simulink model "two_cell_balancing"  (R2024b)
settings: Solver=VariableStepAuto  StartTime=0.0  StopTime=3600  RelTol=1e-3
libraries: simulink x7
settings Model: Creator=nirmithpuneet  LastModifiedBy=nirmithpuneet
settings DebuggingCC: AlgebraicLoopMsg=none

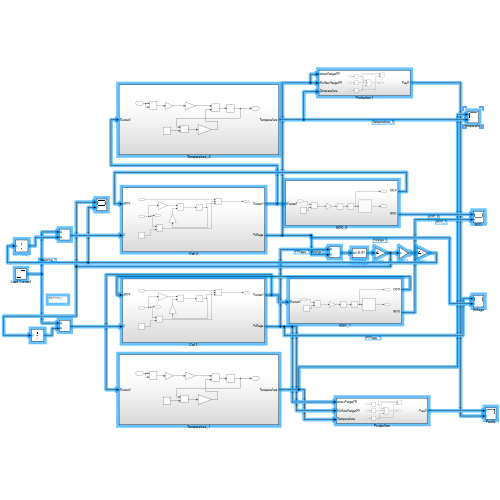
[thumbnail: Simulink's stored preview of the top-level diagram]
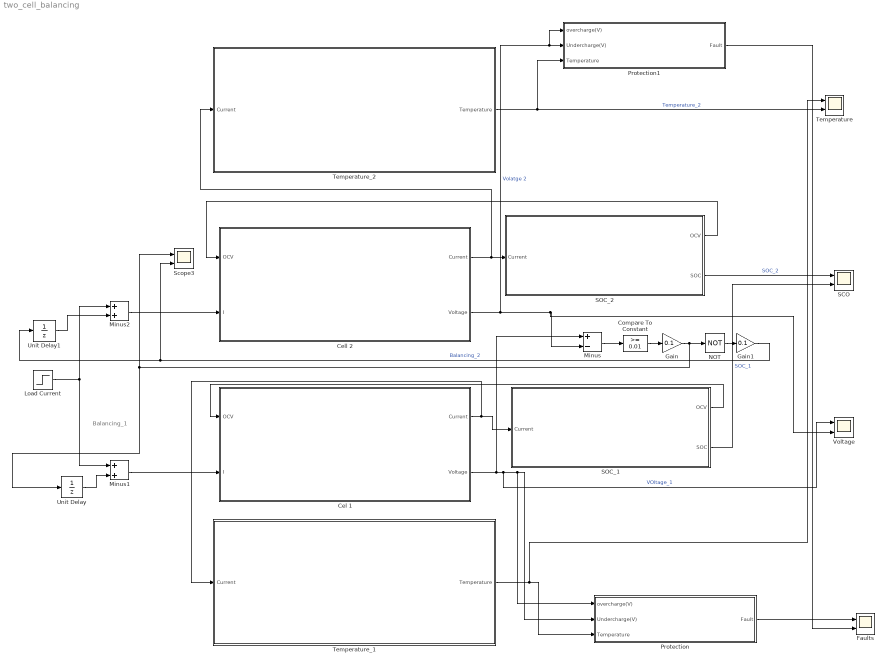
== system two_cell_balancing ==
  note: Balancing_1
  Cel 1 : Subsystem
  Cell 2 : Subsystem
  Compare To Constant : simulink/Logic and Bit Operations/Compare To Constant  relop=>=  const=0.01  OutDataTypeStr=boolean
  Faults : Scope  NumInputPorts=2
  Gain : Gain  Gain=0.1
  Gain1 : Gain  Gain=0.1
  Load Current : Step  After=5  SampleTime=0
  Minus : Sum  Inputs=+-
  Minus1 : Sum
  Minus2 : Sum
  NOT : Logic  Operator=NOT  IconShape=distinctive  AllPortsSameDT=off  OutDataTypeStr=boolean
  Protection : Subsystem
  Protection1 : Subsystem
  SCO : Scope  NumInputPorts=2
  SOC_1 : Subsystem
  SOC_2 : Subsystem
  Scope3 : Scope  NumInputPorts=2
  Temperature : Scope  NumInputPorts=2
  Temperature_1 : Subsystem
  Temperature_2 : Subsystem
  Unit Delay : UnitDelay  SampleTime=-1  HasFrameUpgradeWarning=on
  Unit Delay1 : UnitDelay  SampleTime=-1  HasFrameUpgradeWarning=on
  Voltage : Scope  NumInputPorts=2
  wires:
  Cel 1/1(Current) -> Temperature_1/1(Current), SOC_1/1(Current)
  Cel 1/2(" Voltage") -> Minus/1, Voltage/1, Protection/1(overcharge(V)), Protection/2(Undercharge(V))  "VOltage_1"
  Temperature_1/1(Temperature) -> Temperature/1, Protection/3(Temperature)
  SOC_1/1(OCV) -> Cel 1/1(OCV)
  Cell 2/1(Current) -> Temperature_2/1(Current), SOC_2/1(Current)
  SOC_2/1(OCV) -> Cell 2/1(OCV)
  SOC_2/2(SOC) -> SCO/1  "SOC_2"
  Cell 2/2(" Voltage") -> Protection1/1(overcharge(V)), Protection1/2(Undercharge(V)), Voltage/2, Minus/2  "Volatge 2"
  Minus/1 -> Compare To Constant/1
  Compare To Constant/1 -> Gain/1
  NOT/1 -> Gain1/1
  Load Current/1 -> Minus2/1, Minus1/1
  Minus2/1 -> Cell 2/2(I)
  Minus1/1 -> Cel 1/2(I)
  Gain1/1 -> Unit Delay1/1, Scope3/2  "Balancing_2"
  SOC_1/2(SOC) -> SCO/2  "SOC_1"
  Protection/1(Fault) -> Faults/1
  Gain/1 -> Unit Delay/1, Scope3/1, NOT/1
  Temperature_2/1(Temperature) -> Protection1/3(Temperature), Temperature/2  "Temperature_2"
  Protection1/1(Fault) -> Faults/2
  Unit Delay/1 -> Minus1/2
  Unit Delay1/1 -> Minus2/2

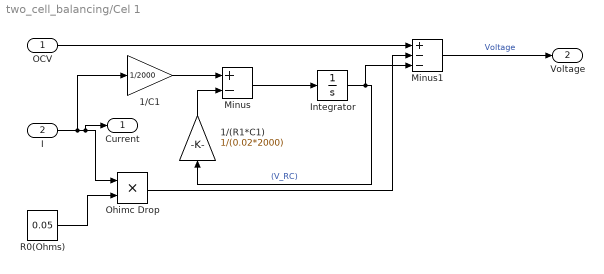
== system two_cell_balancing/Cel 1 ==
  OCV : Inport
  I : Inport  Port=2
  1/(R1*C1) : Gain  Gain=1/(0.02*2000)
  1/C1 : Gain  Gain=1/2000
  Integrator : Integrator
  Minus : Sum  Inputs=+-
  Minus1 : Sum  Inputs=+--
  Ohimc Drop : Product
  R0(Ohms) : Constant  Value=0.05
  Current : Outport
  " Voltage" : Outport  Port=2
  wires:
  Ohimc Drop/1 -> Minus1/2
  1/(R1*C1)/1 -> Minus/2
  Minus/1 -> Integrator/1
  I/1 -> 1/C1/1, Current/1, Ohimc Drop/1
  Minus1/1 -> " Voltage"/1  "Voltage"
  1/C1/1 -> Minus/1
  OCV/1 -> Minus1/1
  R0(Ohms)/1 -> Ohimc Drop/2
  Integrator/1 -> Minus1/3, 1/(R1*C1)/1  "(V_RC)"

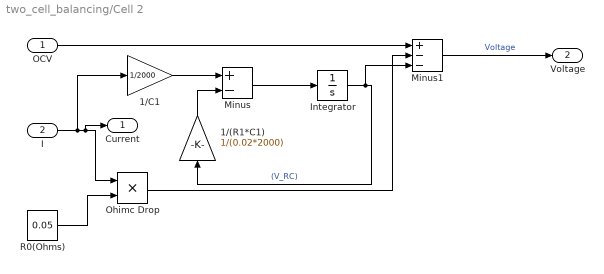
== system two_cell_balancing/Cell 2 ==
  OCV : Inport
  I : Inport  Port=2
  1/(R1*C1) : Gain  Gain=1/(0.02*2000)
  1/C1 : Gain  Gain=1/2000
  Integrator : Integrator
  Minus : Sum  Inputs=+-
  Minus1 : Sum  Inputs=+--
  Ohimc Drop : Product
  R0(Ohms) : Constant  Value=0.05
  Current : Outport
  " Voltage" : Outport  Port=2
  wires:
  Ohimc Drop/1 -> Minus1/2
  1/(R1*C1)/1 -> Minus/2
  Minus/1 -> Integrator/1
  I/1 -> 1/C1/1, Current/1, Ohimc Drop/1
  Minus1/1 -> " Voltage"/1  "Voltage"
  1/C1/1 -> Minus/1
  OCV/1 -> Minus1/1
  R0(Ohms)/1 -> Ohimc Drop/2
  Integrator/1 -> Minus1/3, 1/(R1*C1)/1  "(V_RC)"

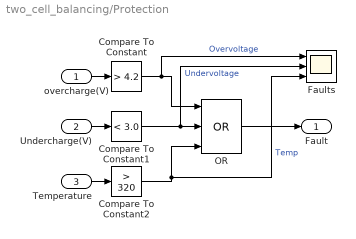
== system two_cell_balancing/Protection ==
  overcharge(V) : Inport
  Undercharge(V) : Inport  Port=2
  Temperature : Inport  Port=3
  Compare To Constant : simulink/Logic and Bit Operations/Compare To Constant  relop=>  const=4.2  OutDataTypeStr=boolean
  Compare To Constant1 : simulink/Logic and Bit Operations/Compare To Constant  relop=<  const=3.0  OutDataTypeStr=boolean
  Compare To Constant2 : simulink/Logic and Bit Operations/Compare To Constant  relop=>  const=320  OutDataTypeStr=boolean
  Faults : Scope  NumInputPorts=3
  OR : Logic  Operator=OR  Inputs=3  IconShape=distinctive  AllPortsSameDT=off  OutDataTypeStr=boolean
  Fault : Outport
  wires:
  Temperature/1 -> Compare To Constant2/1
  Compare To Constant/1 -> Faults/1, OR/1  "Overvoltage"
  Undercharge(V)/1 -> Compare To Constant1/1
  overcharge(V)/1 -> Compare To Constant/1
  Compare To Constant1/1 -> Faults/2, OR/2  "Undervoltage"
  Compare To Constant2/1 -> Faults/3, OR/3  "Temp"
  OR/1 -> Fault/1

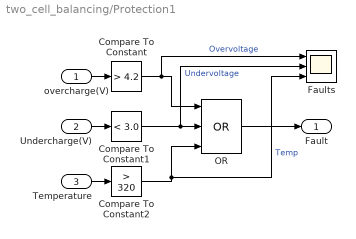
== system two_cell_balancing/Protection1 ==
  overcharge(V) : Inport
  Undercharge(V) : Inport  Port=2
  Temperature : Inport  Port=3
  Compare To Constant : simulink/Logic and Bit Operations/Compare To Constant  relop=>  const=4.2  OutDataTypeStr=boolean
  Compare To Constant1 : simulink/Logic and Bit Operations/Compare To Constant  relop=<  const=3.0  OutDataTypeStr=boolean
  Compare To Constant2 : simulink/Logic and Bit Operations/Compare To Constant  relop=>  const=320  OutDataTypeStr=boolean
  Faults : Scope  NumInputPorts=3
  OR : Logic  Operator=OR  Inputs=3  IconShape=distinctive  AllPortsSameDT=off  OutDataTypeStr=boolean
  Fault : Outport
  wires:
  Temperature/1 -> Compare To Constant2/1
  Compare To Constant/1 -> Faults/1, OR/1  "Overvoltage"
  Undercharge(V)/1 -> Compare To Constant1/1
  overcharge(V)/1 -> Compare To Constant/1
  Compare To Constant1/1 -> Faults/2, OR/2  "Undervoltage"
  Compare To Constant2/1 -> Faults/3, OR/3  "Temp"
  OR/1 -> Fault/1

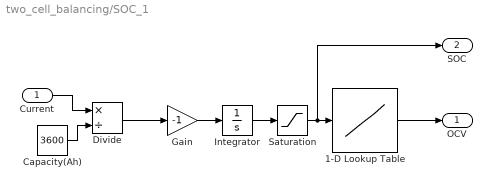
== system two_cell_balancing/SOC_1 ==
  Current : Inport
  1-D Lookup Table : Lookup_n-D  NumberOfTableDimensions=1  BreakpointsForDimension1=[0 0.2 0.5 0.8 1]  Table=[3.0 3.3 3.6 3.9 4.2]  ExtrapMethod=Clip  InternalRulePriority=Speed  RndMeth=Simplest
  Capacity(Ah) : Constant  Value=3600
  Divide : Product  Inputs=*/
  Gain : Gain  Gain=-1
  Integrator : Integrator  InitialCondition=1
  Saturation : Saturate  UpperLimit=1  LowerLimit=0
  OCV : Outport
  SOC : Outport  Port=2
  wires:
  Current/1 -> Divide/1
  Capacity(Ah)/1 -> Divide/2
  Integrator/1 -> Saturation/1
  Gain/1 -> Integrator/1
  Divide/1 -> Gain/1
  Saturation/1 -> SOC/1, 1-D Lookup Table/1
  1-D Lookup Table/1 -> OCV/1

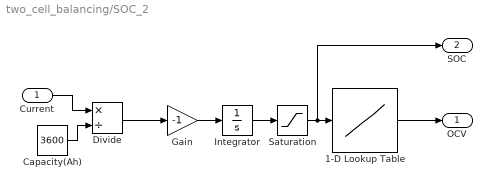
== system two_cell_balancing/SOC_2 ==
  Current : Inport
  1-D Lookup Table : Lookup_n-D  NumberOfTableDimensions=1  BreakpointsForDimension1=[0 0.2 0.5 0.8 1]  Table=[3.0 3.3 3.6 3.9 4.2]  ExtrapMethod=Clip  InternalRulePriority=Speed  RndMeth=Simplest
  Capacity(Ah) : Constant  Value=3600
  Divide : Product  Inputs=*/
  Gain : Gain  Gain=-1
  Integrator : Integrator  InitialCondition=0.9
  Saturation : Saturate  UpperLimit=1  LowerLimit=0
  OCV : Outport
  SOC : Outport  Port=2
  wires:
  Current/1 -> Divide/1
  Capacity(Ah)/1 -> Divide/2
  Integrator/1 -> Saturation/1
  Gain/1 -> Integrator/1
  Divide/1 -> Gain/1
  Saturation/1 -> SOC/1, 1-D Lookup Table/1
  1-D Lookup Table/1 -> OCV/1

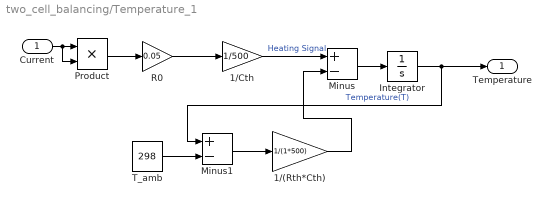
== system two_cell_balancing/Temperature_1 ==
  Current : Inport
  1/(Rth*Cth) : Gain  Gain=1/(1*500)
  1/Cth : Gain  Gain=1/500
  Integrator : Integrator  InitialCondition=298
  Minus : Sum  Inputs=+-
  Minus1 : Sum  Inputs=+-
  Product : Product
  R0 : Gain  Gain=0.05
  T_amb : Constant  Value=298
  Temperature : Outport
  wires:
  Product/1 -> R0/1
  R0/1 -> 1/Cth/1
  Minus/1 -> Integrator/1
  Minus1/1 -> 1/(Rth*Cth)/1
  Current/1 -> Product/2, Product/1
  T_amb/1 -> Minus1/2
  1/Cth/1 -> Minus/1  "Heating Signal"
  Integrator/1 -> Temperature/1, Minus1/1  "Temperature(T)"
  1/(Rth*Cth)/1 -> Minus/2

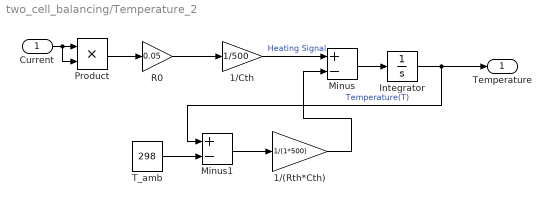
== system two_cell_balancing/Temperature_2 ==
  Current : Inport
  1/(Rth*Cth) : Gain  Gain=1/(1*500)
  1/Cth : Gain  Gain=1/500
  Integrator : Integrator  InitialCondition=298
  Minus : Sum  Inputs=+-
  Minus1 : Sum  Inputs=+-
  Product : Product
  R0 : Gain  Gain=0.05
  T_amb : Constant  Value=298
  Temperature : Outport
  wires:
  Product/1 -> R0/1
  R0/1 -> 1/Cth/1
  Minus/1 -> Integrator/1
  Minus1/1 -> 1/(Rth*Cth)/1
  Current/1 -> Product/2, Product/1
  T_amb/1 -> Minus1/2
  1/Cth/1 -> Minus/1  "Heating Signal"
  Integrator/1 -> Temperature/1, Minus1/1  "Temperature(T)"
  1/(Rth*Cth)/1 -> Minus/2
